simulink model "Test2"  (R2015b)
settings: Solver=FixedStepAuto  StartTime=0.0  StopTime=50  FixedStep=0.01  RelTol=1e-3
undefined symbols (not defined in the file or in its folder): ss2
settings Model: Creator=Druzhinin_Vasily  LastModifiedBy=Druzhinin_Vasily

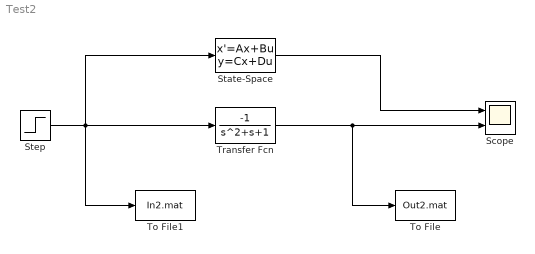
== system Test2 ==
  Scope : Scope  NumInputPorts=2
  State-Space : StateSpace  A=ss2.A  B=ss2.B  C=ss2.C  D=ss2.D  X0=0
  Step : Step  SampleTime=0
  To File : ToFile  Filename=Out2.mat  MatrixName=Out2
  To File1 : ToFile  Filename=In2.mat  MatrixName=In2
  Transfer Fcn : TransferFcn  Numerator=[-1]  Denominator=[ 1 1 1]
  wires:
  Transfer Fcn/1 -> Scope/2, To File/1
  Step/1 -> State-Space/1, Transfer Fcn/1, To File1/1
  State-Space/1 -> Scope/1
